simulink model "SVOC_DFIG"  (R2013a)
settings: Solver=ode15s  StartTime=0.0  StopTime=12  RelTol=1e-3
undefined symbols (not defined in the file): Cdc, Fb, Fs, Fsampling, Grid_Angle_init, Ibase, J_SCIG, Ki, Kp, Lgrid, Llr, Lls, Lm, Ls, Omegamech, P, Qgsc_ref, Qs_ref, Rr, Rs, Sbase, Trated, Ts, Vbase, Vdc_ref, Vp
libraries: powerlib x29, simulink_extras x5, powerlib_extras x5, simulink x4
(part 1 of 2)
settings Model: Creator=Sony  LastModifiedBy=Sony
settings DebuggingCC: UnconnectedInputMsg=none  UnconnectedOutputMsg=none  UnconnectedLineMsg=none

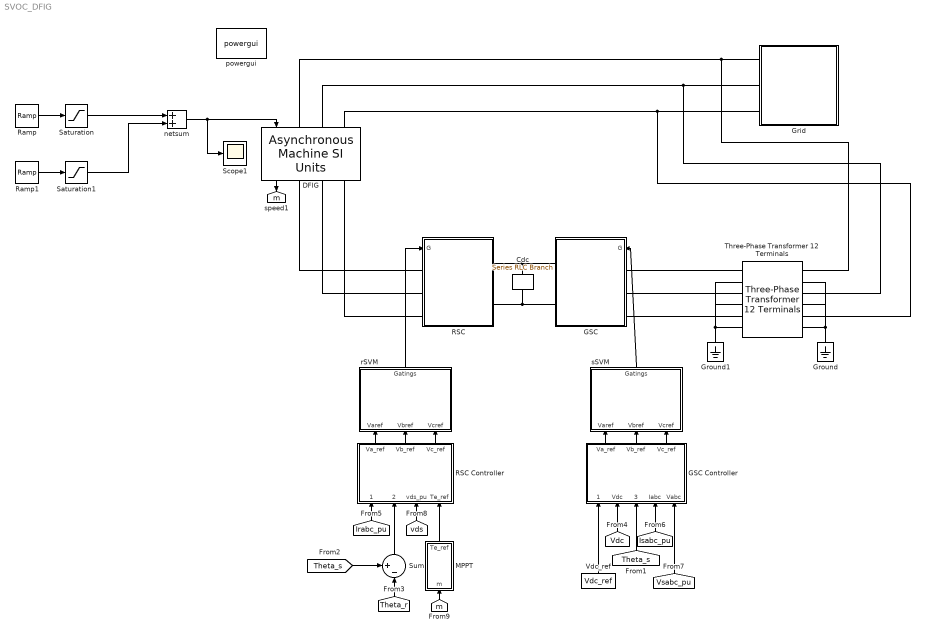
== system SVOC_DFIG ==
  Cdc : powerlib/Elements/Series RLC Branch  LConnTagsString=__new0  RConnTagsString=__new0  BranchType=C  Resistance=1e6  Inductance=1e-3  SetiL0=off  InitialCurrent=0  Capacitance=Cdc  Setx0=on  InitialVoltage=Vdc_ref*Vbase  Measurements=None
  DFIG : powerlib/Machines/Asynchronous Machine SI Units  PresetModel=No  MechanicalLoad=Speed w  ShowDetailedParameters=on  RotorType=Wound  ReferenceFrame=Synchronous  NominalParameters=[Sbase 690 50]  Stator=[Rs Lls]  Rotor=[Rr Llr]  Cage1=[ 0.022 0.226/377]  Cage2=[ 0.022 0.226/377]  Lm=Lm  Mechanical=[J_SCIG 0 P]  PolePairs=2  InitialConditions=[-5.86974e-12 0 317.758 317.758 317.758 -89.9144 150.086 30.0856]  Units=SI  LoadFlowParameters=-0.001  SimulateSaturation=off  Saturation=[0 0;0 0]  TsPowergui=0  TsBlock=-1  IterativeModel=Forward Euler  Pmec=1.5e6
  GSC : Subsystem
  GSC Controller : Subsystem
  Grid : Subsystem
  Ground : powerlib/Elements/Ground  LConnTagsString=a
  Ground1 : powerlib/Elements/Ground  LConnTagsString=a
  MPPT : Subsystem
  RSC : Subsystem
  RSC Controller : Subsystem
  Ramp : simulink/Sources/Ramp  slope=15  start=3  X0=1500*(2*pi/60)
  Ramp1 : simulink/Sources/Ramp  slope=-15  start=6  X0=0
  Saturation : Saturate  UpperLimit=1750*(2*pi/60)  LowerLimit=1225*(2*pi/60)
  Saturation1 : Saturate  UpperLimit=1750*(2*pi/60)  LowerLimit=-(1775-1225)*(2*pi/60)
  Scope1 : Scope
      settings: YMin=-50000  YMax=0  SaveName=ScopeData42
  Sum : Sum  Inputs=+-|
  Three-Phase Transformer 12 Terminals : powerlib/Elements/Three-Phase Transformer 12 Terminals  RatedPower=[ 1.5e6 50 ]  Winding1="[ Vbase*0.358 0.00001  0 ]"  Winding2=[ Vbase 0.00001 0]  RmXm=[ 1e6 1e6 ]
  Vdc_ref : Constant  Value=Vdc_ref
  netsum : Sum  Inputs=2  SaturateOnIntegerOverflow=on  InputSameDT=on  OutDataTypeStr=Inherit: Same as first input
  powergui : powerlib/powergui  Priority=1  SimulationMode=Continuous  SolverType=Tustin  SampleTime=1e-6  frequency=60  SPID=on  DisableSnubberDevices=off  DisableRonSwitches=off  DisableVfSwitches=off  SwTol=0  Interpol=off  DisplayEquations=on  frequencyindice=50  Pbase=1.5e6  ErrMax=1e-4  Iterations=50  UnitsV=kV  UnitsW=MW  FunctionMessages=on  echomessages=off  HookPort=off  EnableUseOfTLC=off  x0status=blocks  RestoreLinks=warning  ResistiveCurrentMeasurement=off  Frange=[0:2:500]  Ylog=off  Xlog=on  ShowGrid=off  save=off  variable=ZData  ZoomFFT=off  StartTime=0.0  cycles=1  DisplayStyle=1  fundamental=60  FreqAxis=off  MaxFrequency=1000  frequencyindicesteady=1  RmsSteady=1  display=off  Ts=0  methode=off
  rSVM : Subsystem
  sSVM : Subsystem
  tag scope: m=global
  wires:
  Vdc_ref/1 -> GSC Controller/1(Vdc_ref)
  [Vdc] -> GSC Controller/2(Vdc)
  GSC Controller/1(Va_ref) -> sSVM/1(Varef)
  GSC Controller/2(Vb_ref) -> sSVM/2(Vbref)
  GSC Controller/3(Vc_ref) -> sSVM/3(Vcref)
  [Theta_s] -> GSC Controller/3(Theta_s)
  sSVM/1(Gatings) -> GSC/1(G)
  rSVM/1(Gatings) -> RSC/1(G)
  RSC Controller/1(Va_ref) -> rSVM/1(Varef)
  RSC Controller/2(Vb_ref) -> rSVM/2(Vbref)
  RSC Controller/3(Vc_ref) -> rSVM/3(Vcref)
  Sum/1 -> RSC Controller/2(Theta_sl)
  [Theta_r] -> Sum/2
  DFIG/1 -> [m]
  [Isabc_pu] -> GSC Controller/4(Iabc)
  [Vsabc_pu] -> GSC Controller/5(Vabc)
  Saturation/1 -> netsum/1
  [Irabc_pu] -> RSC Controller/1(Irabc_pu)
  [vds] -> RSC Controller/3(vds_pu)
  MPPT/1(Te_ref) -> RSC Controller/4(Te_ref)
  [m] -> MPPT/1(m)
  [Theta_s] -> Sum/1
  Ramp/1 -> Saturation/1
  Ramp1/1 -> Saturation1/1
  Saturation1/1 -> netsum/2
  netsum/1 -> Scope1/1, DFIG/1
  connections:
  Grid/LConn1 -- DFIG/LConn1 -- Three-Phase Transformer 12 Terminals/RConn1
  Grid/LConn3 -- DFIG/LConn3 -- Three-Phase Transformer 12 Terminals/RConn5
  Grid/LConn2 -- DFIG/LConn2 -- Three-Phase Transformer 12 Terminals/RConn3
  RSC/LConn1 -- DFIG/RConn1
  RSC/LConn2 -- DFIG/RConn2
  RSC/LConn3 -- DFIG/RConn3
  GSC/RConn1 -- Cdc/LConn1 -- RSC/RConn1
  GSC/RConn2 -- Cdc/RConn1 -- RSC/RConn2
  GSC/LConn1 -- Three-Phase Transformer 12 Terminals/LConn1
  GSC/LConn2 -- Three-Phase Transformer 12 Terminals/LConn3
  GSC/LConn3 -- Three-Phase Transformer 12 Terminals/LConn5
  Three-Phase Transformer 12 Terminals/RConn6 -- Three-Phase Transformer 12 Terminals/RConn2 -- Three-Phase Transformer 12 Terminals/RConn4 -- Ground/LConn1
  Three-Phase Transformer 12 Terminals/LConn6 -- Three-Phase Transformer 12 Terminals/LConn2 -- Three-Phase Transformer 12 Terminals/LConn4 -- Ground1/LConn1

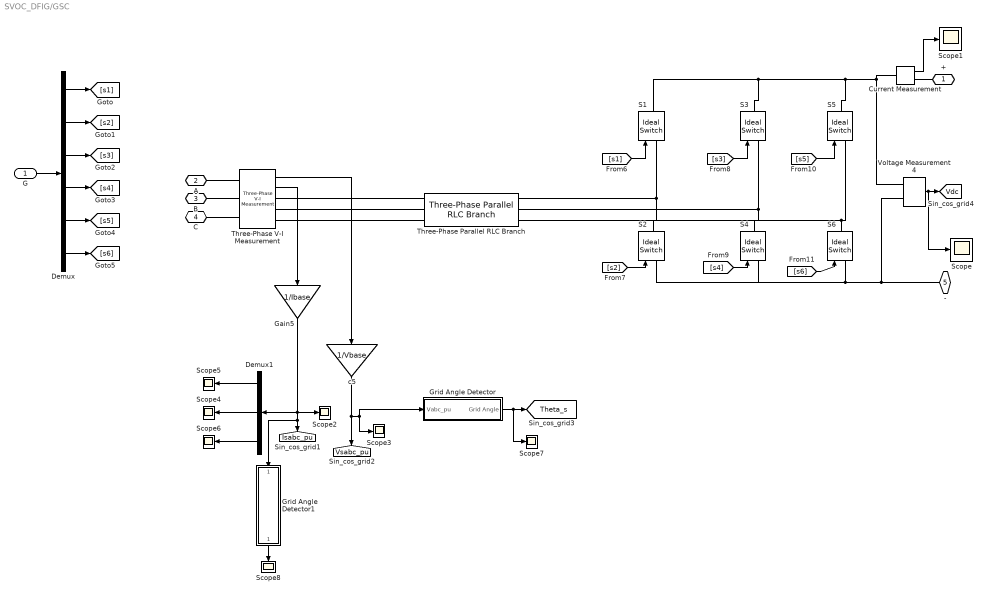
== system SVOC_DFIG/GSC ==
  G : Inport
  " S1" : powerlib/Power Electronics/Ideal Switch  Ron=Ron  Lon=0  IC=1  Rs=inf  Cs=inf  Measurements=off
  " S2" : powerlib/Power Electronics/Ideal Switch  Ron=Ron  Lon=0  IC=0  Rs=inf  Cs=inf  Measurements=off
  " S3" : powerlib/Power Electronics/Ideal Switch  Ron=Ron  Lon=0  IC=1  Rs=inf  Cs=inf  Measurements=off
  " S4" : powerlib/Power Electronics/Ideal Switch  Ron=Ron  Lon=0  IC=0  Rs=inf  Cs=inf  Measurements=off
  " S5" : powerlib/Power Electronics/Ideal Switch  Ron=Ron  Lon=0  IC=1  Rs=inf  Cs=inf  Measurements=off
  " S6" : powerlib/Power Electronics/Ideal Switch  Ron=Ron  Lon=0  IC=0  Rs=inf  Cs=inf  Measurements=off
  Current Measurement : powerlib/Measurements/Current Measurement  PhasorSimulation=off  OutputType=Complex  PSBequivalent=0
  Demux : Demux  Outputs=6
  Demux1 : Demux  Outputs=3
  Gain5 : Gain  Gain=1/Ibase
  Grid Angle Detector : Subsystem
  Grid Angle Detector1 : Subsystem
  Scope{,1..8} (9 alike) : Scope
      Scope settings: YMin=0  YMax=600  SaveName=ScopeData8
      Scope1 settings: YMin=-225  YMax=200  SaveName=ScopeData9
      Scope2 settings: YMin=-50  YMax=50  SaveName=ScopeData33
      Scope3 settings: SaveName=ScopeData32
      Scope4 settings: SaveName=ScopeData14
      Scope5 settings: YMin=-2000  YMax=2500  SaveName=ScopeData39
      Scope6 settings: SaveName=ScopeData19
      Scope7 settings: YMin=0  YMax=6.5  SaveName=ScopeData27
      Scope8 settings: YMin=0  YMax=6.5  SaveName=ScopeData54
  Three-Phase Parallel RLC Branch : powerlib/Elements/Three-Phase Parallel RLC Branch  LConnTagsString=A|B|C  RConnTagsString=A|B|C  BranchType=L  Resistance=inf  Inductance=Lgrid  Capacitance=1e-6  Measurements=None
  Three-Phase V-I Measurement : powerlib/Measurements/Three-Phase V-I Measurement  VoltageMeasurement=phase-to-ground  SetLabelV=off  LabelV=Vabc  Vpu=off  VpuLL=off  CurrentMeasurement=yes  SetLabelI=off  LabelI=Iabc  Ipu=off  Pbase=100e6  Vbase=500e3  OutputType=Complex  PhasorSimulation=off  PSBequivalent=0
  Voltage Measurement4 : powerlib/Measurements/Voltage Measurement  PhasorSimulation=off  OutputType=Complex  PSBequivalent=0
  c5 : Gain  Gain=1/Vbase
  + : PMIOPort  Port=1  Side=Right
  A : PMIOPort  Port=2  Side=Left
  B : PMIOPort  Port=3  Side=Left
  C : PMIOPort  Port=4  Side=Left
  - : PMIOPort  Port=5  Side=Right
  tag scope: Isabc_pu=global, Theta_s=global, Vdc=global, Vsabc_pu=global
  wires:
  [s1] -> " S1"/1
  [s5] -> " S5"/1
  Demux/1 -> [s1]
  Demux/2 -> [s2]
  Demux/3 -> [s3]
  Demux/4 -> [s4]
  Demux/5 -> [s5]
  Demux/6 -> [s6]
  G/1 -> Demux/1
  [s3] -> " S3"/1
  Grid Angle Detector/1(Grid Angle) -> Scope7/1, [Theta_s]
  Voltage Measurement4/1 -> Scope/1, [Vdc]
  [s6] -> " S6"/1
  [s4] -> " S4"/1
  [s2] -> " S2"/1
  Gain5/1 -> Scope2/1, Grid Angle Detector1/1(Vabc_pu), [Isabc_pu], Demux1/1
  c5/1 -> Scope3/1, Grid Angle Detector/1(Vabc_pu), [Vsabc_pu]
  Demux1/1 -> Scope5/1
  Demux1/2 -> Scope4/1
  Demux1/3 -> Scope6/1
  Current Measurement/1 -> Scope1/1
  Grid Angle Detector1/1(Grid Angle) -> Scope8/1
  Three-Phase V-I Measurement/1 -> c5/1
  Three-Phase V-I Measurement/2 -> Gain5/1
  connections:
  Voltage Measurement4/LConn1 -- Current Measurement/LConn1 -- " S5"/RConn1 -- " S3"/RConn1 -- " S1"/RConn1
  " S2"/RConn1 -- " S1"/LConn1 -- Three-Phase Parallel RLC Branch/RConn1
  " S4"/RConn1 -- " S3"/LConn1 -- Three-Phase Parallel RLC Branch/RConn2
  -/RConn1 -- Voltage Measurement4/LConn2 -- " S2"/LConn1 -- " S4"/LConn1 -- " S6"/LConn1
  A/RConn1 -- Three-Phase V-I Measurement/LConn1
  B/RConn1 -- Three-Phase V-I Measurement/LConn2
  C/RConn1 -- Three-Phase V-I Measurement/LConn3
  " S6"/RConn1 -- " S5"/LConn1 -- Three-Phase Parallel RLC Branch/RConn3
  Current Measurement/RConn1 -- +/RConn1
  Three-Phase Parallel RLC Branch/LConn1 -- Three-Phase V-I Measurement/RConn1
  Three-Phase Parallel RLC Branch/LConn2 -- Three-Phase V-I Measurement/RConn2
  Three-Phase Parallel RLC Branch/LConn3 -- Three-Phase V-I Measurement/RConn3

== system SVOC_DFIG/GSC Controller ==
  Vdc_ref : Inport
  Vdc : Inport  Port=2
  Theta_s : Inport  Port=3
  Iabc : Inport  Port=4
  Vabc : Inport  Port=5
  Add : Sum  Inputs=+-
  Add1 : Sum  Inputs=-+-
  Add2 : Sum  Inputs=-++
  Constant : Constant  Value=Qgsc_ref
  Mux6 : Mux  Inputs=2
  Product1 : Product  Inputs=*/
  Scope{1,3..5} (4 alike) : Scope  NumInputPorts=4
      Scope1 settings: YMin=0.506283~-1~-3~-3  YMax=0.506296~1~2.5~3  SaveName=ScopeData47
      Scope3 settings: YMin=1.04021~1.04021~-3~-6.05  YMax=1.14971~1.14971~3~-5.75  SaveName=ScopeData23
      Scope4 settings: YMin=-27.475~-75~-90~890  YMax=-27.275~75~40~1020  SaveName=ScopeData38
      Scope5 settings: YMin=-1~-20~-20~-2.5  YMax=1~20~20~2  SaveName=ScopeData43
  Sum : Sum  Inputs=|+-
  Sum2 : Sum  Inputs=|+-
  Vdc_Ctr1 : powerlib_extras/Discrete  Control Blocks/Discrete PI Controller  Kp=Kp  Ki=Ki  Par_Limits=[1e6 -1e6]  Init=0  Ts=50e-6
  Xl1 : Subsystem
  Xl2 : Subsystem
  abc/dq : Subsystem
  abc/dq1 : Subsystem
  constant2 : Gain  Gain=(1/Vbase)
  constant5 : Gain  Gain=-1.5
  dq/abc : Subsystem
  id_Ctr1 : powerlib_extras/Discrete  Control Blocks/Discrete PI Controller  Kp=Kp  Ki=Ki  Par_Limits=[1e6 -1e6]  Init=0  Ts=50e-6
  iq_Ctr2 : powerlib_extras/Discrete  Control Blocks/Discrete PI Controller  Kp=Kp  Ki=Ki  Par_Limits=[1e6 -1e6]  Init=0  Ts=50e-6
  Va_ref : Outport
  Vb_ref : Outport  Port=2
  Vc_ref : Outport  Port=3
  tag scope: vds=global
  wires:
  Vdc_ref/1 -> Scope3/1, Add/1
  Add/1 -> Vdc_Ctr1/1, Scope3/3
  constant5/1 -> Product1/2
  Constant/1 -> Product1/1
  dq/abc/1(Va) -> Va_ref/1
  dq/abc/2(Vb) -> Vb_ref/1
  dq/abc/3(Vc) -> Vc_ref/1
  Mux6/1 -> dq/abc/1(vdq)
  id_Ctr1/1 -> Scope4/4, Add2/1
  Sum/1 -> Scope4/3, id_Ctr1/1
  abc/dq/2(Vqg) -> Scope1/2, Add1/2
  abc/dq/1(Vdg) -> Add2/2, constant5/1, Scope1/1, [vds]
  Sum2/1 -> Scope5/3, iq_Ctr2/1
  Xl2/1(Out1) -> Add1/3
  Theta_s/1 -> abc/dq1/2(Theta), abc/dq/2(Theta), dq/abc/2(Theta)
  Xl1/1(Out1) -> Add2/3
  Iabc/1 -> abc/dq1/1(Iabc)
  Vabc/1 -> abc/dq/1(Vabc)
  Add2/1 -> Mux6/1
  Add1/1 -> Mux6/2
  constant2/1 -> Scope3/2, Add/2
  abc/dq1/1(Idg) -> Scope1/3, Xl2/1(In1), Scope4/2, Sum/2
  Product1/1 -> Scope5/1, Sum2/1
  abc/dq1/2(Iqg) -> Xl1/1(In1), Scope1/4, Scope5/2, Sum2/2
  Vdc_Ctr1/1 -> Scope4/1, Sum/1, Scope3/4
  iq_Ctr2/1 -> Scope5/4, Add1/1
  Vdc/1 -> constant2/1

== system SVOC_DFIG/Grid ==
  AC Voltage Source1 : powerlib/Electrical Sources/AC Voltage Source  Amplitude=Vp  Phase=-120+Grid_Angle_init  Frequency=50  SampleTime=0  Measurements=None
  AC Voltage Source2 : powerlib/Electrical Sources/AC Voltage Source  Amplitude=Vp  Phase=-240+Grid_Angle_init  Frequency=50  SampleTime=0  Measurements=None
  AC Voltage Source3 : powerlib/Electrical Sources/AC Voltage Source  Amplitude=Vp  Phase=0+Grid_Angle_init  Frequency=50  SampleTime=0  Measurements=None
  Demux1 : Demux  Outputs=3
  Demux2 : Demux  Outputs=3
  Gain5 : Gain  Gain=1/Ibase
  Grid Angle Detector : Subsystem
  Ground : powerlib/Elements/Ground  LConnTagsString=a
  Scope{1..10} (10 alike) : Scope
      Scope1 settings: YMin=-0.35  YMax=0.025  SaveName=ScopeData36
      Scope2 settings: YMin=-50  YMax=50  SaveName=ScopeData21
      Scope3 settings: YMin=-1.5  YMax=1.5  SaveName=ScopeData35
      Scope4 settings: SaveName=ScopeData48
      Scope5 settings: SaveName=ScopeData49
      Scope6 settings: YMin=-15  YMax=15  SaveName=ScopeData50
      Scope7 settings: SaveName=ScopeData51
      Scope8 settings: SaveName=ScopeData52
      Scope9 settings: YMin=-1.5  YMax=1.5  SaveName=ScopeData53
  Three-Phase V-I Measurement : powerlib/Measurements/Three-Phase V-I Measurement  VoltageMeasurement=phase-to-ground  SetLabelV=off  LabelV=Vabc  Vpu=off  VpuLL=off  CurrentMeasurement=yes  SetLabelI=off  LabelI=Iabc  Ipu=off  Pbase=100e6  Vbase=500e3  OutputType=Complex  PhasorSimulation=off  PSBequivalent=0
  c5 : Gain  Gain=1/Vbase
  Phase A : PMIOPort  Port=1  Side=Left
  Phase B : PMIOPort  Port=2  Side=Left
  Phase C : PMIOPort  Port=3  Side=Left
  tag scope: iag=global, vag=global
  wires:
  Grid Angle Detector/1(Grid Angle) -> Scope1/1
  Gain5/1 -> Demux1/1, Scope2/1
  Three-Phase V-I Measurement/2 -> Gain5/1
  Three-Phase V-I Measurement/1 -> Grid Angle Detector/1(Vabc_pu), c5/1, Scope3/1
  Demux1/1 -> [iag], Scope6/1
  Demux1/2 -> Scope5/1
  Demux1/3 -> Scope7/1
  c5/1 -> Demux2/1, Scope4/1
  Demux2/1 -> [vag], Scope9/1
  Demux2/2 -> Scope8/1
  Demux2/3 -> Scope10/1
  connections:
  Three-Phase V-I Measurement/LConn1 -- AC Voltage Source3/RConn1
  Three-Phase V-I Measurement/LConn3 -- AC Voltage Source2/RConn1
  AC Voltage Source2/LConn1 -- AC Voltage Source3/LConn1 -- AC Voltage Source1/LConn1 -- Ground/LConn1
  Phase A/RConn1 -- Three-Phase V-I Measurement/RConn1
  Phase B/RConn1 -- Three-Phase V-I Measurement/RConn2
  Phase C/RConn1 -- Three-Phase V-I Measurement/RConn3
  AC Voltage Source1/RConn1 -- Three-Phase V-I Measurement/LConn2

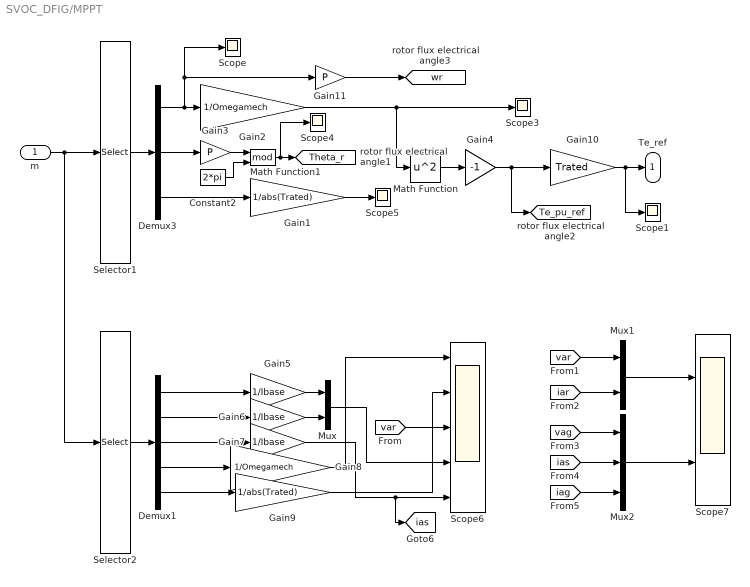
== system SVOC_DFIG/MPPT ==
  m : Inport
  Constant2 : Constant  Value=2*pi
  Demux1 : Demux  Outputs=5
  Demux3 : Demux  Outputs=3
  Gain1 : Gain  Gain=1/abs(Trated)
  Gain10 : Gain  Gain=Trated
  Gain11 : Gain  Gain=P
  Gain2 : Gain  Gain=1/Omegamech  SampleTime=1/Fsampling
  Gain3 : Gain  Gain=P
  Gain4 : Gain  Gain=-1
  Gain5 : Gain  Gain=1/Ibase
  Gain6 : Gain  Gain=1/Ibase
  Gain7 : Gain  Gain=1/Ibase
  Gain8 : Gain  Gain=1/Omegamech  SampleTime=1/Fsampling
  Gain9 : Gain  Gain=1/abs(Trated)
  Math Function : Math  Operator=square  SaturateOnIntegerOverflow=on
  Math Function1 : Math  Operator=mod  SampleTime=1/Fsampling  SaturateOnIntegerOverflow=on
  Mux : Mux  Inputs=2
  Mux1 : Mux  Inputs=2
  Mux2 : Mux  Inputs=3
  Scope{,1,3..5} (5 alike) : Scope
      Scope settings: YMin=127.5  YMax=185  SaveName=ScopeData4
      Scope1 settings: YMin=-9010.65  YMax=-3010.65  SaveName=ScopeData7
      Scope3 settings: YMin=0.4  YMax=1.2  SaveName=ScopeData15
      Scope4 settings: YMin=0  YMax=6.5  SaveName=ScopeData17
      Scope5 settings: YMin=-10  YMax=10  SaveName=ScopeData18
  Scope6 : Scope  NumInputPorts=5
      settings: YMin=0.6~-5~-1.25~-5~-5  YMax=1.2~5~1.25~5~5  SaveName=ScopeData28
  Scope7 : Scope  NumInputPorts=2
      settings: YMin=-2~-2  YMax=2~2  SaveName=ScopeData55
  Selector1 : Selector  InputPortWidth=22  IndexOptions=Index vector (dialog)  Indices=[20 22 21]  OutputSizes=1
  Selector2 : Selector  InputPortWidth=22  IndexOptions=Index vector (dialog)  Indices=[1 2 11 20 21]  OutputSizes=1
  Te_ref : Outport
  tag scope: Te_pu_ref=global, Theta_r=global, ias=global, wr=global
  wires:
  Demux3/3 -> Gain1/1
  Selector1/1 -> Demux3/1
  Gain2/1 -> Math Function/1, Scope3/1
  Constant2/1 -> Math Function1/2
  Demux3/2 -> Gain3/1
  Math Function/1 -> Gain4/1
  Gain10/1 -> Scope1/1, Te_ref/1
  Gain3/1 -> Math Function1/1
  Math Function1/1 -> Scope4/1, [Theta_r]
  Gain1/1 -> Scope5/1
  Selector2/1 -> Demux1/1
  m/1 -> Selector2/1, Selector1/1
  Demux1/1 -> Gain5/1
  Demux1/2 -> Gain6/1
  Demux1/3 -> Gain7/1
  Demux1/4 -> Gain8/1
  Demux1/5 -> Gain9/1
  Gain4/1 -> [Te_pu_ref], Gain10/1
  Gain7/1 -> [ias], Scope6/5
  Gain5/1 -> Mux/1
  Gain6/1 -> Mux/2
  Mux/1 -> Scope6/4
  [var] -> Scope6/3
  Gain8/1 -> Scope6/1
  Gain9/1 -> Scope6/2
  Mux1/1 -> Scope7/1
  Mux2/1 -> Scope7/2
  Demux3/1 -> Scope/1, Gain11/1, Gain2/1
  Gain11/1 -> [wr]
  [var] -> Mux1/1
  [iar] -> Mux1/2
  [ias] -> Mux2/2
  [iag] -> Mux2/3
  [vag] -> Mux2/1

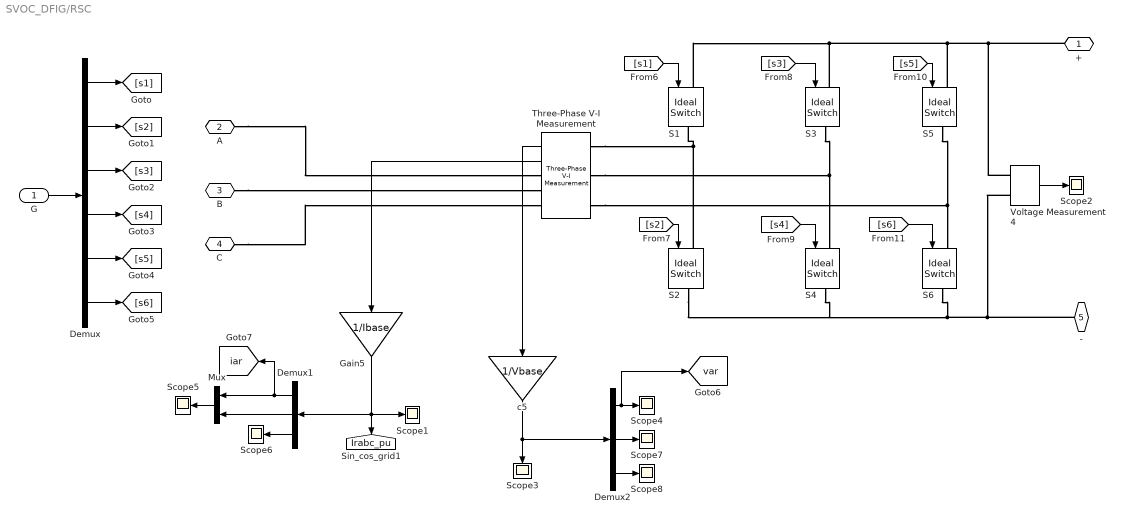
== system SVOC_DFIG/RSC ==
  G : Inport
  " S1" : powerlib/Power Electronics/Ideal Switch  Ron=Ron  Lon=0  IC=1  Rs=inf  Cs=inf  Measurements=off
  " S2" : powerlib/Power Electronics/Ideal Switch  Ron=Ron  Lon=0  IC=0  Rs=inf  Cs=inf  Measurements=off
  " S3" : powerlib/Power Electronics/Ideal Switch  Ron=Ron  Lon=0  IC=1  Rs=inf  Cs=inf  Measurements=off
  " S4" : powerlib/Power Electronics/Ideal Switch  Ron=Ron  Lon=0  IC=0  Rs=inf  Cs=inf  Measurements=off
  " S5" : powerlib/Power Electronics/Ideal Switch  Ron=Ron  Lon=0  IC=1  Rs=inf  Cs=inf  Measurements=off
  " S6" : powerlib/Power Electronics/Ideal Switch  Ron=Ron  Lon=0  IC=0  Rs=inf  Cs=inf  Measurements=off
  Demux : Demux  Outputs=6
  Demux1 : Demux  Outputs=3
  Demux2 : Demux  Outputs=3
  Gain5 : Gain  Gain=1/Ibase
  Mux : Mux  Inputs=2
  Scope{1..8} (8 alike) : Scope
      Scope1 settings: YMin=-25  YMax=22.5  SaveName=ScopeData31
      Scope2 settings: YMin=0  YMax=570.102
      Scope3 settings: YMin=-2  YMax=2  SaveName=ScopeData30
      Scope4 settings: YMin=-2  YMax=2  SaveName=ScopeData41
      Scope5 settings: YMin=-15  YMax=15  SaveName=ScopeData40
      Scope6 settings: SaveName=ScopeData20
      Scope7 settings: SaveName=ScopeData24
      Scope8 settings: SaveName=ScopeData25
  Three-Phase V-I Measurement : powerlib/Measurements/Three-Phase V-I Measurement  VoltageMeasurement=phase-to-ground  SetLabelV=off  LabelV=Vabc  Vpu=off  VpuLL=off  CurrentMeasurement=yes  SetLabelI=off  LabelI=Iabc  Ipu=off  Pbase=100e6  Vbase=500e3  OutputType=Complex  PhasorSimulation=off  PSBequivalent=0
  Voltage Measurement4 : powerlib/Measurements/Voltage Measurement  PhasorSimulation=off  OutputType=Complex  PSBequivalent=0
  c5 : Gain  Gain=1/Vbase
  + : PMIOPort  Port=1  Side=Right
  A : PMIOPort  Port=2  Side=Left
  B : PMIOPort  Port=3  Side=Left
  C : PMIOPort  Port=4  Side=Left
  - : PMIOPort  Port=5  Side=Right
  tag scope: Irabc_pu=global, iar=global, var=global
  wires:
  [s1] -> " S1"/1
  [s5] -> " S5"/1
  Demux/1 -> [s1]
  Demux/2 -> [s2]
  Demux/3 -> [s3]
  Demux/4 -> [s4]
  Demux/5 -> [s5]
  Demux/6 -> [s6]
  G/1 -> Demux/1
  [s2] -> " S2"/1
  [s3] -> " S3"/1
  [s4] -> " S4"/1
  [s6] -> " S6"/1
  Voltage Measurement4/1 -> Scope2/1
  Three-Phase V-I Measurement/1 -> c5/1
  Gain5/1 -> Scope1/1, [Irabc_pu], Demux1/1
  Demux1/1 -> [iar], Mux/1
  Demux1/2 -> Mux/2
  Mux/1 -> Scope5/1
  c5/1 -> Demux2/1, Scope3/1
  Demux2/1 -> [var], Scope4/1
  Demux1/3 -> Scope6/1
  Demux2/2 -> Scope7/1
  Demux2/3 -> Scope8/1
  Three-Phase V-I Measurement/2 -> Gain5/1
  connections:
  +/RConn1 -- Voltage Measurement4/LConn1 -- " S5"/LConn1 -- " S3"/LConn1 -- " S1"/LConn1
  " S2"/LConn1 -- " S1"/RConn1 -- Three-Phase V-I Measurement/LConn1
  " S3"/RConn1 -- " S4"/LConn1 -- Three-Phase V-I Measurement/LConn2
  " S5"/RConn1 -- " S6"/LConn1 -- Three-Phase V-I Measurement/LConn3
  -/RConn1 -- Voltage Measurement4/LConn2 -- " S2"/RConn1 -- " S4"/RConn1 -- " S6"/RConn1
  A/RConn1 -- Three-Phase V-I Measurement/RConn1
  B/RConn1 -- Three-Phase V-I Measurement/RConn2
  C/RConn1 -- Three-Phase V-I Measurement/RConn3

== system SVOC_DFIG/RSC Controller ==
  note: actual value
  Irabc_pu : Inport
  Theta_sl : Inport  Port=2
  vds_pu : Inport  Port=3
  Te_ref : Inport  Port=4
  Gain : Gain  Gain=(2*Ls*Qs_ref)/(3*Lm)
  Gain1 : Gain  Gain=1/(2*pi*Fb*Lm)
  Gain2 : Gain  Gain=-(2*2*pi*Fb*Ls)/(3*P*Lm)
  Gain3 : Gain  Gain=Vbase
  Gain4 : Gain  Gain=1/Ibase
  Gain5 : Gain  Gain=1/Ibase
  Math Function : Math  Operator=reciprocal  SaturateOnIntegerOverflow=on
  Math Function1 : Math  Operator=reciprocal  SaturateOnIntegerOverflow=on
  Multiply : Product
  Scope2 : Scope  NumInputPorts=4
      settings: YMin=-1~-1~-1~-0.5  YMax=1~1~1~1.25  SaveName=ScopeData44
  Scope3 : Scope  NumInputPorts=4
      settings: YMin=2.56425~2.51~-0.03~-0.005  YMax=2.56433~2.59~0.05~0.055  SaveName=ScopeData16
  Sum1 : Sum  Inputs=-+|
  Sum2 : Sum  Inputs=-+|
  Sum3 : Sum  Inputs=-+|
  abc/dq1 : Subsystem
  dq/abc : Subsystem
  id_Ctr1 : powerlib_extras/Discrete  Control Blocks/Discrete PI Controller  Kp=Kp  Ki=Ki  Par_Limits=[1e6 -1e6]  Init=0  Ts=50e-6
  id_Ctr2 : powerlib_extras/Discrete  Control Blocks/Discrete PI Controller  Kp=Kp  Ki=Ki  Par_Limits=[1e6 -1e6]  Init=0  Ts=50e-6
  Va_ref : Outport
  Vb_ref : Outport  Port=2
  Vc_ref : Outport  Port=3
  wires:
  dq/abc/3(Vcr_ref) -> Vc_ref/1
  Sum1/1 -> id_Ctr2/1, Scope2/3
  Math Function1/1 -> Gain2/1
  Sum2/1 -> Scope3/3, id_Ctr1/1
  Gain3/1 -> Gain1/1, Math Function1/1, Math Function/1
  dq/abc/2(Vbr_ref) -> Vb_ref/1
  id_Ctr2/1 -> Scope2/4, dq/abc/2(vq_ref)
  Gain1/1 -> Sum3/1
  id_Ctr1/1 -> Scope3/4, dq/abc/1(vd_ref)
  Gain/1 -> Sum3/2
  Math Function/1 -> Gain/1
  Te_ref/1 -> Multiply/2
  Gain2/1 -> Multiply/1
  Irabc_pu/1 -> abc/dq1/1(Irabc)
  dq/abc/1(Var_ref) -> Va_ref/1
  Theta_sl/1 -> abc/dq1/2(Theta_sl), dq/abc/3(Theta_sl)
  abc/dq1/1(Idr) -> Scope3/2, Sum2/1
  abc/dq1/2(Iqr) -> Scope2/2, Sum1/1
  Gain5/1 -> Sum2/2, Scope3/1
  Gain4/1 -> Sum1/2, Scope2/1
  vds_pu/1 -> Gain3/1
  Sum3/1 -> Gain4/1
  Multiply/1 -> Gain5/1

== system SVOC_DFIG/rSVM ==
  Varef : Inport
  Vbref : Inport  Port=2
  Vcref : Inport  Port=3
  Add : Sum
  Cartesian to Polar : simulink_extras/Transformations/Cartesian to Polar
  Constant : Constant  Value=2*pi
  Constant1 : Constant  Value=2*pi
  Divide : Product  Inputs=/*
  Dwell Time Calculator : Subsystem
  Math Function : Math  Operator=rem  SaturateOnIntegerOverflow=on
  Mux7 : Mux  Inputs=3
  Pulses : Subsystem
  Saturation : Saturate  UpperLimit=1  LowerLimit=0.01  SampleTime=1/Fsampling
  Sector judge : Subsystem
  Ts : Constant  Value=Ts
  Zero-Order Hold : ZeroOrderHold  SampleTime=Ts/2
  Zero-Order Hold1 : ZeroOrderHold  SampleTime=Ts/2
  abc/alphabeta : Subsystem
  constant : Gain  Gain=3^0.5
  constant2 : Gain  Gain=(1/Vbase)
  ma : Scope
      settings: SaveName=ScopeData5
  theta : Scope
      settings: YMin=0  YMax=6.5  SaveName=ScopeData6
  Gatings : Outport
  wires:
  Dwell Time Calculator/3(T0) -> Pulses/4(T0)
  constant/1 -> Divide/2
  Pulses/1(Gating) -> Gatings/1
  Cartesian to Polar/1 -> constant/1
  Divide/1 -> Saturation/1
  Ts/1 -> Dwell Time Calculator/3(Ts)
  Varef/1 -> Mux7/1
  Dwell Time Calculator/1(Ta) -> Pulses/2(Ta1)
  Dwell Time Calculator/2(Tb) -> Pulses/3(Tb1)
  Sector judge/2(Cal_theta) -> Dwell Time Calculator/1(Theta)
  Saturation/1 -> Zero-Order Hold/1, ma/1
  Zero-Order Hold/1 -> Dwell Time Calculator/2(ma)
  Zero-Order Hold1/1 -> Sector judge/1(theta), theta/1
  Sector judge/1(Sector) -> Pulses/1(Sector)
  abc/alphabeta/1(Valpha) -> Cartesian to Polar/1
  Mux7/1 -> abc/alphabeta/1(Vabc)
  Vbref/1 -> Mux7/2
  abc/alphabeta/2(Vbeta) -> Cartesian to Polar/2
  Vcref/1 -> Mux7/3
  Cartesian to Polar/2 -> Add/1
  Math Function/1 -> Zero-Order Hold1/1
  Constant/1 -> Add/2
  Add/1 -> Math Function/1
  Constant1/1 -> Math Function/2
  constant2/1 -> Divide/1
  [Vdc] -> constant2/1

== system SVOC_DFIG/sSVM ==
  Varef : Inport
  Vbref : Inport  Port=2
  Vcref : Inport  Port=3
  Add : Sum
  Cartesian to Polar : simulink_extras/Transformations/Cartesian to Polar
  Constant : Constant  Value=2*pi
  Constant1 : Constant  Value=2*pi
  Divide : Product  Inputs=/*
  Dwell Time Calculator : Subsystem
  Math Function : Math  Operator=rem  SaturateOnIntegerOverflow=on
  Mux7 : Mux  Inputs=3
  Pulses : Subsystem
  Saturation : Saturate  UpperLimit=1  LowerLimit=0.01  SampleTime=1/Fsampling
  Scope{,1..3} (4 alike) : Scope
      Scope settings: YMin=0  YMax=8  SaveName=ScopeData10
      Scope1 settings: YMin=25  YMax=350  SaveName=ScopeData37
      Scope2 settings: YMin=0  YMax=8  SaveName=ScopeData45
      Scope3 settings: YMin=-0.01  YMax=0.01  SaveName=ScopeData46
  Sector judge : Subsystem
  Ts : Constant  Value=Ts
  Zero-Order Hold : ZeroOrderHold  SampleTime=Ts/2
  Zero-Order Hold1 : ZeroOrderHold  SampleTime=Ts/2
  abc/alphabeta : Subsystem
  constant : Gain  Gain=3^0.5
  constant2 : Gain  Gain=(1/Vbase)
  ma : Scope
      settings: YMin=0  YMax=2  SaveName=ScopeData5
  theta : Scope
      settings: YMin=0  YMax=6.5  SaveName=ScopeData6
  Gatings : Outport
  wires:
  Dwell Time Calculator/3(T0) -> Pulses/4(T0)
  constant/1 -> Scope1/1, Divide/2
  Pulses/1(Gating) -> Gatings/1
  Cartesian to Polar/1 -> constant/1
  Divide/1 -> Scope3/1, Saturation/1
  Ts/1 -> Dwell Time Calculator/3(Ts)
  Varef/1 -> Mux7/1
  Dwell Time Calculator/1(Ta) -> Pulses/2(Ta1)
  Dwell Time Calculator/2(Tb) -> Pulses/3(Tb1)
  Sector judge/2(Cal_theta) -> Dwell Time Calculator/1(Theta)
  Saturation/1 -> Zero-Order Hold/1, ma/1
  Zero-Order Hold/1 -> Dwell Time Calculator/2(ma)
  constant2/1 -> Scope2/1, Divide/1
  Zero-Order Hold1/1 -> Sector judge/1(theta), theta/1
  Sector judge/1(Sector) -> Scope/1, Pulses/1(Sector)
  abc/alphabeta/1(Valpha) -> Cartesian to Polar/1
  Mux7/1 -> abc/alphabeta/1(Vabc)
  Vbref/1 -> Mux7/2
  abc/alphabeta/2(Vbeta) -> Cartesian to Polar/2
  Vcref/1 -> Mux7/3
  Cartesian to Polar/2 -> Add/1
  Math Function/1 -> Zero-Order Hold1/1
  Constant/1 -> Add/2
  Add/1 -> Math Function/1
  Constant1/1 -> Math Function/2
  [Vdc] -> constant2/1

== system SVOC_DFIG/GSC/Grid Angle Detector ==
  Vabc_pu : Inport
  Add : Sum
  Beta1 : Fcn  Expr=(1/(3^.5))*(u(1)+2*u(2))
  Cartesian to Polar1 : simulink_extras/Transformations/Cartesian to Polar
  Constant : Constant  Value=2*pi
  Math Function : Math  Operator=rem  SaturateOnIntegerOverflow=on
  Scope3 : Scope  NumInputPorts=2
      settings: YMin=-1~-5  YMax=2~5  SaveName=ScopeData34
  Scope5 : Scope
      settings: SaveName=ScopeData13
  alpha1 : Fcn  Expr=u(1)
  Grid Angle : Outport
  wires:
  Beta1/1 -> Scope3/2, Cartesian to Polar1/2
  Vabc_pu/1 -> alpha1/1, Beta1/1
  Math Function/1 -> Grid Angle/1
  alpha1/1 -> Scope3/1, Cartesian to Polar1/1
  Cartesian to Polar1/2 -> Add/1
  Constant/1 -> Math Function/2, Add/2
  Add/1 -> Math Function/1
  Cartesian to Polar1/1 -> Scope5/1

== system SVOC_DFIG/GSC/Grid Angle Detector1 ==
  Vabc_pu : Inport
  Add : Sum
  Beta1 : Fcn  Expr=(1/(3^.5))*(u(1)+2*u(2))
  Cartesian to Polar1 : simulink_extras/Transformations/Cartesian to Polar
  Constant : Constant  Value=2*pi
  Math Function : Math  Operator=rem  SaturateOnIntegerOverflow=on
  Scope3 : Scope  NumInputPorts=2
      settings: YMin=-1~-5  YMax=2~5  SaveName=ScopeData34
  Scope5 : Scope
      settings: SaveName=ScopeData13
  alpha1 : Fcn  Expr=u(1)
  Grid Angle : Outport
  wires:
  Beta1/1 -> Scope3/2, Cartesian to Polar1/2
  Vabc_pu/1 -> alpha1/1, Beta1/1
  Math Function/1 -> Grid Angle/1
  alpha1/1 -> Scope3/1, Cartesian to Polar1/1
  Cartesian to Polar1/2 -> Add/1
  Constant/1 -> Math Function/2, Add/2
  Add/1 -> Math Function/1
  Cartesian to Polar1/1 -> Scope5/1

== system SVOC_DFIG/GSC Controller/Xl1 ==
  In1 : Inport
  Constant1 : Constant  Value=2*pi*50
  Constant2 : Constant  Value=0
  Gain : Gain  Gain=Lgrid/Vbase
  Matrix Multiply : Product
  netsum : Sum  Inputs=-+  SaturateOnIntegerOverflow=on  InputSameDT=on  OutDataTypeStr=Inherit: Same as first input
  Out1 : Outport
  wires:
  In1/1 -> Matrix Multiply/1
  Matrix Multiply/1 -> Gain/1
  Constant2/1 -> netsum/1
  Constant1/1 -> netsum/2
  netsum/1 -> Matrix Multiply/2
  Gain/1 -> Out1/1

== system SVOC_DFIG/GSC Controller/Xl2 ==
  In1 : Inport
  Constant1 : Constant  Value=2*pi*50
  Constant2 : Constant  Value=0
  Gain : Gain  Gain=Lgrid/Vbase
  Matrix Multiply : Product
  netsum : Sum  Inputs=-+  SaturateOnIntegerOverflow=on  InputSameDT=on  OutDataTypeStr=Inherit: Same as first input
  Out1 : Outport
  wires:
  In1/1 -> Matrix Multiply/1
  Matrix Multiply/1 -> Gain/1
  Constant1/1 -> netsum/2
  netsum/1 -> Matrix Multiply/2
  Gain/1 -> Out1/1
  Constant2/1 -> netsum/1

== system SVOC_DFIG/GSC Controller/abc//dq ==
  Vabc : Inport
  Theta : Inport  Port=2
  Add{,1,3..4} (4 alike) : Sum  Inputs=+-
  Add2 : Sum  Inputs=+++
  Add5 : Sum  Inputs=+++
  Constant : Constant  Value=(2*pi)/3
  Constant1 : Constant  Value=(4*pi)/3
  Constant2 : Constant  Value=(2*pi)/3
  Constant3 : Constant  Value=(4*pi)/3
  Demux2 : Demux  Outputs=3
  Gain : Gain  Gain=2/3
  Gain1 : Gain  Gain=-(2/3)*0
  Product{1..6} (6 alike) : Product
  Scope5 : Scope  NumInputPorts=4
      settings: YMin=1.41421~-1~-1~-1  YMax=1.41421~1~1~1  SaveName=ScopeData26
  Trigonometric Function : Trigonometry  Operator=cos
  Trigonometric Function1 : Trigonometry  Operator=cos
  Trigonometric Function2 : Trigonometry  Operator=cos
  Trigonometric Function3 : Trigonometry
  Trigonometric Function4 : Trigonometry
  Trigonometric Function5 : Trigonometry
  Vdg : Outport
  Vqg : Outport  Port=2
  wires:
  Trigonometric Function1/1 -> Product2/1
  Constant/1 -> Add/2
  Trigonometric Function/1 -> Product1/1
  Trigonometric Function2/1 -> Product3/1
  Add/1 -> Trigonometric Function1/1
  Constant1/1 -> Add1/2
  Product2/1 -> Add2/2
  Product1/1 -> Add2/1
  Constant2/1 -> Add3/2
  Demux2/1 -> Product4/2, Product1/2
  Product5/1 -> Add5/2
  Constant3/1 -> Add4/2
  Add4/1 -> Trigonometric Function5/1
  Trigonometric Function3/1 -> Product4/1
  Trigonometric Function4/1 -> Product5/1
  Add3/1 -> Trigonometric Function4/1
  Trigonometric Function5/1 -> Product6/1
  Demux2/2 -> Product5/2, Product2/2
  Demux2/3 -> Product6/2, Product3/2
  Product4/1 -> Add5/1
  Add5/1 -> Gain1/1
  Product6/1 -> Add5/3
  Add1/1 -> Trigonometric Function2/1
  Product3/1 -> Add2/3
  Theta/1 -> Add/1, Trigonometric Function/1, Add1/1, Add4/1, Add3/1, Trigonometric Function3/1
  Vabc/1 -> Demux2/1
  Gain/1 -> Scope5/1, Vdg/1
  Add2/1 -> Gain/1
  Gain1/1 -> Scope5/2, Vqg/1

== system SVOC_DFIG/GSC Controller/abc//dq1 ==
  Iabc : Inport
  Theta : Inport  Port=2
  Add{,1,3..4} (4 alike) : Sum  Inputs=+-
  Add2 : Sum  Inputs=+++
  Add5 : Sum  Inputs=+++
  Constant : Constant  Value=(2*pi)/3
  Constant1 : Constant  Value=(4*pi)/3
  Constant2 : Constant  Value=(2*pi)/3
  Constant3 : Constant  Value=(4*pi)/3
  Demux2 : Demux  Outputs=3
  Gain : Gain  Gain=2/3
  Gain1 : Gain  Gain=-2/3
  Product{1..6} (6 alike) : Product
  Trigonometric Function : Trigonometry  Operator=cos
  Trigonometric Function1 : Trigonometry  Operator=cos
  Trigonometric Function2 : Trigonometry  Operator=cos
  Trigonometric Function3 : Trigonometry
  Trigonometric Function4 : Trigonometry
  Trigonometric Function5 : Trigonometry
  Idg : Outport
  Iqg : Outport  Port=2
  wires:
  Trigonometric Function1/1 -> Product2/1
  Constant/1 -> Add/2
  Trigonometric Function/1 -> Product1/1
  Trigonometric Function2/1 -> Product3/1
  Add/1 -> Trigonometric Function1/1
  Constant1/1 -> Add1/2
  Product2/1 -> Add2/2
  Product1/1 -> Add2/1
  Constant2/1 -> Add3/2
  Demux2/1 -> Product4/2, Product1/2
  Product5/1 -> Add5/2
  Constant3/1 -> Add4/2
  Add4/1 -> Trigonometric Function5/1
  Trigonometric Function3/1 -> Product4/1
  Trigonometric Function4/1 -> Product5/1
  Add3/1 -> Trigonometric Function4/1
  Trigonometric Function5/1 -> Product6/1
  Demux2/2 -> Product5/2, Product2/2
  Demux2/3 -> Product6/2, Product3/2
  Product4/1 -> Add5/1
  Add5/1 -> Gain1/1
  Product6/1 -> Add5/3
  Add1/1 -> Trigonometric Function2/1
  Product3/1 -> Add2/3
  Theta/1 -> Add/1, Trigonometric Function/1, Add1/1, Add4/1, Add3/1, Trigonometric Function3/1
  Gain1/1 -> Iqg/1
  Iabc/1 -> Demux2/1
  Gain/1 -> Idg/1
  Add2/1 -> Gain/1

== system SVOC_DFIG/GSC Controller/dq//abc ==
  vdq : Inport
  Theta : Inport  Port=2
  Add{,1..6} (7 alike) : Sum  Inputs=+-
  Constant : Constant  Value=(2*pi)/3
  Constant1 : Constant  Value=(4*pi)/3
  Constant2 : Constant  Value=(2*pi)/3
  Constant3 : Constant  Value=(4*pi)/3
  Demux2 : Demux  Outputs=2
  Product{1..6} (6 alike) : Product
  Trigonometric Function : Trigonometry  Operator=cos
  Trigonometric Function1 : Trigonometry  Operator=cos
  Trigonometric Function2 : Trigonometry  Operator=cos
  Trigonometric Function3 : Trigonometry
  Trigonometric Function4 : Trigonometry
  Trigonometric Function5 : Trigonometry
  Va : Outport
  Vb : Outport  Port=2
  Vc : Outport  Port=3
  wires:
  Trigonometric Function1/1 -> Product2/1
  Constant/1 -> Add/2
  Trigonometric Function/1 -> Product1/1
  Add/1 -> Trigonometric Function1/1
  Product1/1 -> Add2/1
  Constant2/1 -> Add3/2
  Demux2/1 -> Product1/2, Product2/2, Product3/2
  Trigonometric Function3/1 -> Product4/1
  Trigonometric Function4/1 -> Product5/1
  Add3/1 -> Trigonometric Function4/1
  vdq/1 -> Demux2/1
  Add2/1 -> Va/1
  Product4/1 -> Add2/2
  Demux2/2 -> Product4/2, Product6/2, Product5/2
  Product2/1 -> Add6/1
  Add6/1 -> Vb/1
  Product5/1 -> Add6/2
  Trigonometric Function2/1 -> Product3/1
  Constant1/1 -> Add1/2
  Add1/1 -> Trigonometric Function2/1
  Constant3/1 -> Add4/2
  Trigonometric Function5/1 -> Product6/1
  Add4/1 -> Trigonometric Function5/1
  Theta/1 -> Trigonometric Function/1, Trigonometric Function3/1, Add/1, Add4/1, Add1/1, Add3/1
  Product3/1 -> Add5/1
  Add5/1 -> Vc/1
  Product6/1 -> Add5/2

== system SVOC_DFIG/Grid/Grid Angle Detector ==
  Vabc_pu : Inport
  Add : Sum
  Beta1 : Fcn  Expr=(1/(3^.5))*(u(1)+2*u(2))
  Cartesian to Polar1 : simulink_extras/Transformations/Cartesian to Polar
  Constant : Constant  Value=2*pi
  Math Function : Math  Operator=rem  SaturateOnIntegerOverflow=on
  Scope5 : Scope
      settings: SaveName=ScopeData11
  alpha1 : Fcn  Expr=u(1)
  Grid Angle : Outport
  wires:
  Beta1/1 -> Cartesian to Polar1/2
  Vabc_pu/1 -> alpha1/1, Beta1/1
  Math Function/1 -> Grid Angle/1
  alpha1/1 -> Cartesian to Polar1/1
  Cartesian to Polar1/2 -> Add/1
  Constant/1 -> Math Function/2, Add/2
  Add/1 -> Math Function/1
  Cartesian to Polar1/1 -> Scope5/1

== system SVOC_DFIG/RSC Controller/abc//dq1 ==
  Irabc : Inport
  Theta_sl : Inport  Port=2
  Add{,1,3..4} (4 alike) : Sum  Inputs=+-
  Add2 : Sum  Inputs=+++
  Add5 : Sum  Inputs=+++
  Constant : Constant  Value=(2*pi)/3
  Constant1 : Constant  Value=(4*pi)/3
  Constant2 : Constant  Value=(2*pi)/3
  Constant3 : Constant  Value=(4*pi)/3
  Demux2 : Demux  Outputs=3
  Gain : Gain  Gain=2/3
  Gain1 : Gain  Gain=-2/3
  Product{1..6} (6 alike) : Product
  Trigonometric Function : Trigonometry  Operator=cos
  Trigonometric Function1 : Trigonometry  Operator=cos
  Trigonometric Function2 : Trigonometry  Operator=cos
  Trigonometric Function3 : Trigonometry
  Trigonometric Function4 : Trigonometry
  Trigonometric Function5 : Trigonometry
  Idr : Outport
  Iqr : Outport  Port=2
  wires:
  Trigonometric Function1/1 -> Product2/1
  Constant/1 -> Add/2
  Trigonometric Function/1 -> Product1/1
  Trigonometric Function2/1 -> Product3/1
  Add/1 -> Trigonometric Function1/1
  Constant1/1 -> Add1/2
  Product2/1 -> Add2/2
  Product1/1 -> Add2/1
  Constant2/1 -> Add3/2
  Demux2/1 -> Product4/2, Product1/2
  Product5/1 -> Add5/2
  Constant3/1 -> Add4/2
  Add4/1 -> Trigonometric Function5/1
  Trigonometric Function3/1 -> Product4/1
  Trigonometric Function4/1 -> Product5/1
  Add3/1 -> Trigonometric Function4/1
  Trigonometric Function5/1 -> Product6/1
  Demux2/2 -> Product5/2, Product2/2
  Demux2/3 -> Product6/2, Product3/2
  Product4/1 -> Add5/1
  Add5/1 -> Gain1/1
  Product6/1 -> Add5/3
  Add1/1 -> Trigonometric Function2/1
  Product3/1 -> Add2/3
  Theta_sl/1 -> Add/1, Trigonometric Function/1, Add1/1, Add4/1, Add3/1, Trigonometric Function3/1
  Gain1/1 -> Iqr/1
  Irabc/1 -> Demux2/1
  Gain/1 -> Idr/1
  Add2/1 -> Gain/1

== system SVOC_DFIG/RSC Controller/dq//abc ==
  vd_ref : Inport
  vq_ref : Inport  Port=2
  Theta_sl : Inport  Port=3
  Add{,1..6} (7 alike) : Sum  Inputs=+-
  Constant : Constant  Value=(2*pi)/3
  Constant1 : Constant  Value=(4*pi)/3
  Constant2 : Constant  Value=(2*pi)/3
  Constant3 : Constant  Value=(4*pi)/3
  Product{1..6} (6 alike) : Product
  Trigonometric Function : Trigonometry  Operator=cos
  Trigonometric Function1 : Trigonometry  Operator=cos
  Trigonometric Function2 : Trigonometry  Operator=cos
  Trigonometric Function3 : Trigonometry
  Trigonometric Function4 : Trigonometry
  Trigonometric Function5 : Trigonometry
  Var_ref : Outport
  Vbr_ref : Outport  Port=2
  Vcr_ref : Outport  Port=3
  wires:
  Trigonometric Function1/1 -> Product2/1
  Constant/1 -> Add/2
  Trigonometric Function/1 -> Product1/1
  Add/1 -> Trigonometric Function1/1
  Product1/1 -> Add2/1
  Constant2/1 -> Add3/2
  vd_ref/1 -> Product1/2, Product2/2, Product3/2
  Trigonometric Function3/1 -> Product4/1
  Trigonometric Function4/1 -> Product5/1
  Add3/1 -> Trigonometric Function4/1
  Add2/1 -> Var_ref/1
  Product4/1 -> Add2/2
  vq_ref/1 -> Product4/2, Product6/2, Product5/2
  Product2/1 -> Add6/1
  Add6/1 -> Vbr_ref/1
  Product5/1 -> Add6/2
  Trigonometric Function2/1 -> Product3/1
  Constant1/1 -> Add1/2
  Add1/1 -> Trigonometric Function2/1
  Constant3/1 -> Add4/2
  Trigonometric Function5/1 -> Product6/1
  Add4/1 -> Trigonometric Function5/1
  Theta_sl/1 -> Trigonometric Function/1, Trigonometric Function3/1, Add/1, Add4/1, Add1/1, Add3/1
  Product3/1 -> Add5/1
  Add5/1 -> Vcr_ref/1
  Product6/1 -> Add5/2

== system SVOC_DFIG/rSVM/Dwell Time Calculator ==
  Theta : Inport
  ma : Inport  Port=2
  Ts : Inport  Port=3
  Add : Sum  Inputs=--+
  Compare To Zero : simulink/Logic and Bit Operations/Compare To Zero  relop=>=  OutDataTypeStr=boolean
  Data Type Conversion : DataTypeConversion  OutDataTypeStr=double
  Mux : Mux  Inputs=3
  Product : Product  RndMeth=Zero
  Scope : Scope  NumInputPorts=3
      settings: YMin=0~0~-2.71051e-20  YMax=0.0001~0.0001~0.000425  SaveName=ScopeData12
  cTa : Fcn  Expr=u(2)*u(3)*sin((pi/3)-u(1))
  cTb : Fcn  Expr=u(2)*u(3)*sin(u(1))
  Ta : Outport
  Tb : Outport  Port=2
  T0 : Outport  Port=3
  wires:
  Product/1 -> Scope/1, T0/1
  Theta/1 -> Mux/1
  ma/1 -> Mux/2
  Ts/1 -> Add/3, Mux/3
  Mux/1 -> cTb/1, cTa/1
  Add/1 -> Product/2, Compare To Zero/1
  Data Type Conversion/1 -> Product/1
  Compare To Zero/1 -> Data Type Conversion/1
  cTa/1 -> Scope/2, Ta/1, Add/1
  cTb/1 -> Scope/3, Tb/1, Add/2

== system SVOC_DFIG/rSVM/Pulses ==
  Sector : Inport
  Ta1 : Inport  Port=2
  Tb1 : Inport  Port=3
  T0 : Inport  Port=4
  Data Type Conversion : DataTypeConversion  OutDataTypeStr=boolean
  Data Type Conversion1 : DataTypeConversion  OutDataTypeStr=boolean
  Data Type Conversion2 : DataTypeConversion  OutDataTypeStr=boolean
  Inverter Leg a : Subsystem
  Inverter Leg b : Subsystem
  Inverter Leg c : Subsystem
  Logical Operator : Logic  Operator=NOT  AllPortsSameDT=off
  Logical Operator1 : Logic  Operator=NOT  AllPortsSameDT=off
  Logical Operator2 : Logic  Operator=NOT  AllPortsSameDT=off
  Mux : Mux  Inputs=6
  Scope1 : Scope
      settings: SaveName=ScopeData2
  Scope3 : Scope
      settings: YMin=0  YMax=8  SaveName=ScopeData22
  Sector Select a : MultiPortSwitch  Inputs=6  DiagnosticForDefault=None
  Sector Select b : MultiPortSwitch  Inputs=6  DiagnosticForDefault=None
  Sector Select c : MultiPortSwitch  Inputs=6  DiagnosticForDefault=None
  Switching Segment Calculator : Subsystem
  Gating : Outport
  wires:
  Sector/1 -> Sector Select a/1, Scope1/1, Sector Select b/1, Sector Select c/1
  Data Type Conversion2/1 -> Logical Operator/1, Mux/1
  Data Type Conversion1/1 -> Logical Operator1/1, Mux/3
  Data Type Conversion/1 -> Logical Operator2/1, Mux/5
  Mux/1 -> Gating/1
  Logical Operator/1 -> Mux/2
  Logical Operator1/1 -> Mux/4
  Logical Operator2/1 -> Mux/6
  Switching Segment Calculator/1(Segment) -> Scope3/1, Inverter Leg c/1(Segment), Inverter Leg a/1(Segment), Inverter Leg b/1(Segment)
  T0/1 -> Switching Segment Calculator/1(T0)
  Ta1/1 -> Switching Segment Calculator/2(Ta)
  Tb1/1 -> Switching Segment Calculator/3(Tb)
  Inverter Leg a/1(Out1) -> Sector Select a/2
  Inverter Leg a/2(Out2) -> Sector Select a/3
  Inverter Leg a/3(Out3) -> Sector Select a/4
  Inverter Leg a/4(Out4) -> Sector Select a/5
  Inverter Leg a/5(Out5) -> Sector Select a/6
  Inverter Leg a/6(Out6) -> Sector Select a/7
  Inverter Leg b/1(Out1) -> Sector Select b/2
  Inverter Leg b/2(Out2) -> Sector Select b/3
  Inverter Leg b/3(Out3) -> Sector Select b/4
  Inverter Leg b/4(Out4) -> Sector Select b/5
  Inverter Leg b/5(Out5) -> Sector Select b/6
  Inverter Leg b/6(Out6) -> Sector Select b/7
  Inverter Leg c/1(Out1) -> Sector Select c/2
  Inverter Leg c/2(Out2) -> Sector Select c/3
  Inverter Leg c/3(Out3) -> Sector Select c/4
  Inverter Leg c/4(Out4) -> Sector Select c/5
  Inverter Leg c/5(Out5) -> Sector Select c/6
  Inverter Leg c/6(Out6) -> Sector Select c/7
  Sector Select c/1 -> Data Type Conversion/1
  Sector Select b/1 -> Data Type Conversion1/1
  Sector Select a/1 -> Data Type Conversion2/1

== system SVOC_DFIG/rSVM/Sector judge ==
  theta : Inport
  Add : Sum
  Constant : Constant  Value=2*pi
  Constant1 : Constant  OutDataTypeStr=boolean
  Constant2 : Constant  Value=2*pi
  Gain1 : Gain  Gain=3/pi
  Gain2 : Gain  Gain=pi/3
  Math Function1 : Math  Operator=rem  SaturateOnIntegerOverflow=on
  Rounding Function : Rounding
  Sum1 : Sum  Inputs=|++  SaturateOnIntegerOverflow=on
  Sum2 : Sum  Inputs=|-+
  Sector : Outport
  Cal_theta : Outport  Port=2
  wires:
  Gain1/1 -> Rounding Function/1
  Rounding Function/1 -> Gain2/1, Sum1/1
  Sum1/1 -> Sector/1
  Constant1/1 -> Sum1/2
  Gain2/1 -> Sum2/1
  Sum2/1 -> Cal_theta/1
  theta/1 -> Add/1
  Math Function1/1 -> Sum2/2, Gain1/1
  Constant/1 -> Add/2
  Add/1 -> Math Function1/1
  Constant2/1 -> Math Function1/2

== system SVOC_DFIG/rSVM/abc//alphabeta ==
  Vabc : Inport
  Beta1 : Fcn  Expr=(1/(3^.5))*(u(1)+2*u(2))
  alpha1 : Fcn  Expr=u(1)
  Valpha : Outport
  Vbeta : Outport  Port=2
  wires:
  Vabc/1 -> Beta1/1, alpha1/1
  alpha1/1 -> Valpha/1
  Beta1/1 -> Vbeta/1

== system SVOC_DFIG/sSVM/Dwell Time Calculator ==
  Theta : Inport
  ma : Inport  Port=2
  Ts : Inport  Port=3
  Add : Sum  Inputs=--+
  Compare To Zero : simulink/Logic and Bit Operations/Compare To Zero  relop=>=  OutDataTypeStr=boolean
  Data Type Conversion : DataTypeConversion  OutDataTypeStr=double
  Mux : Mux  Inputs=3
  Product : Product  RndMeth=Zero
  Scope : Scope  NumInputPorts=3
      settings: YMin=-5~-5~-5  YMax=5~5~5  SaveName=ScopeData12
  cTa : Fcn  Expr=u(2)*u(3)*sin((pi/3)-u(1))
  cTb : Fcn  Expr=u(2)*u(3)*sin(u(1))
  Ta : Outport
  Tb : Outport  Port=2
  T0 : Outport  Port=3
  wires:
  Product/1 -> Scope/1, T0/1
  Theta/1 -> Mux/1
  ma/1 -> Mux/2
  Ts/1 -> Add/3, Mux/3
  Mux/1 -> cTb/1, cTa/1
  Add/1 -> Product/2, Compare To Zero/1
  Data Type Conversion/1 -> Product/1
  Compare To Zero/1 -> Data Type Conversion/1
  cTa/1 -> Scope/2, Ta/1, Add/1
  cTb/1 -> Scope/3, Tb/1, Add/2

== system SVOC_DFIG/sSVM/Pulses ==
  Sector : Inport
  Ta1 : Inport  Port=2
  Tb1 : Inport  Port=3
  T0 : Inport  Port=4
  Data Type Conversion : DataTypeConversion  OutDataTypeStr=boolean
  Data Type Conversion1 : DataTypeConversion  OutDataTypeStr=boolean
  Data Type Conversion2 : DataTypeConversion  OutDataTypeStr=boolean
  Inverter Leg a : Subsystem
  Inverter Leg b : Subsystem
  Inverter Leg c : Subsystem
  Logical Operator : Logic  Operator=NOT  AllPortsSameDT=off
  Logical Operator1 : Logic  Operator=NOT  AllPortsSameDT=off
  Logical Operator2 : Logic  Operator=NOT  AllPortsSameDT=off
  Mux : Mux  Inputs=6
  Scope1 : Scope
      settings: SaveName=ScopeData2
  Scope3 : Scope
      settings: YMin=0  YMax=8  SaveName=ScopeData29
  Sector Select a : MultiPortSwitch  Inputs=6  DiagnosticForDefault=None
  Sector Select b : MultiPortSwitch  Inputs=6  DiagnosticForDefault=None
  Sector Select c : MultiPortSwitch  Inputs=6  DiagnosticForDefault=None
  Switching Segment Calculator : Subsystem
  Gating : Outport
  wires:
  Sector/1 -> Sector Select a/1, Scope1/1, Sector Select b/1, Sector Select c/1
  Data Type Conversion/1 -> Logical Operator/1, Mux/1
  Data Type Conversion1/1 -> Logical Operator1/1, Mux/3
  Data Type Conversion2/1 -> Logical Operator2/1, Mux/5
  Mux/1 -> Gating/1
  Logical Operator/1 -> Mux/2
  Logical Operator1/1 -> Mux/4
  Logical Operator2/1 -> Mux/6
  Switching Segment Calculator/1(Segment) -> Inverter Leg c/1(Segment), Inverter Leg a/1(Segment), Scope3/1, Inverter Leg b/1(Segment)
  T0/1 -> Switching Segment Calculator/1(T0)
  Ta1/1 -> Switching Segment Calculator/2(Ta)
  Tb1/1 -> Switching Segment Calculator/3(Tb)
  Inverter Leg a/1(Out1) -> Sector Select a/2
  Inverter Leg a/2(Out2) -> Sector Select a/3
  Inverter Leg a/3(Out3) -> Sector Select a/4
  Inverter Leg a/4(Out4) -> Sector Select a/5
  Inverter Leg a/5(Out5) -> Sector Select a/6
  Inverter Leg a/6(Out6) -> Sector Select a/7
  Inverter Leg b/1(Out1) -> Sector Select b/2
  Inverter Leg b/2(Out2) -> Sector Select b/3
  Inverter Leg b/3(Out3) -> Sector Select b/4
  Inverter Leg b/4(Out4) -> Sector Select b/5
  Inverter Leg b/5(Out5) -> Sector Select b/6
  Inverter Leg b/6(Out6) -> Sector Select b/7
  Inverter Leg c/1(Out1) -> Sector Select c/2
  Inverter Leg c/2(Out2) -> Sector Select c/3
  Inverter Leg c/3(Out3) -> Sector Select c/4
  Inverter Leg c/4(Out4) -> Sector Select c/5
  Inverter Leg c/5(Out5) -> Sector Select c/6
  Inverter Leg c/6(Out6) -> Sector Select c/7
  Sector Select a/1 -> Data Type Conversion/1
  Sector Select b/1 -> Data Type Conversion1/1
  Sector Select c/1 -> Data Type Conversion2/1

== system SVOC_DFIG/sSVM/Sector judge ==
  theta : Inport
  Add : Sum
  Constant : Constant  Value=2*pi
  Constant1 : Constant  OutDataTypeStr=boolean
  Constant2 : Constant  Value=2*pi
  Gain1 : Gain  Gain=3/pi
  Gain2 : Gain  Gain=pi/3
  Math Function1 : Math  Operator=rem  SaturateOnIntegerOverflow=on
  Rounding Function : Rounding
  Sum1 : Sum  Inputs=|++  SaturateOnIntegerOverflow=on
  Sum2 : Sum  Inputs=|-+
  Sector : Outport
  Cal_theta : Outport  Port=2
  wires:
  Gain1/1 -> Rounding Function/1
  Rounding Function/1 -> Gain2/1, Sum1/1
  Sum1/1 -> Sector/1
  Constant1/1 -> Sum1/2
  Gain2/1 -> Sum2/1
  Sum2/1 -> Cal_theta/1
  theta/1 -> Add/1
  Math Function1/1 -> Sum2/2, Gain1/1
  Constant/1 -> Add/2
  Add/1 -> Math Function1/1
  Constant2/1 -> Math Function1/2

== system SVOC_DFIG/sSVM/abc//alphabeta ==
  Vabc : Inport
  Beta1 : Fcn  Expr=(1/(3^.5))*(u(1)+2*u(2))
  alpha1 : Fcn  Expr=u(1)
  Valpha : Outport
  Vbeta : Outport  Port=2
  wires:
  Vabc/1 -> Beta1/1, alpha1/1
  alpha1/1 -> Valpha/1
  Beta1/1 -> Vbeta/1

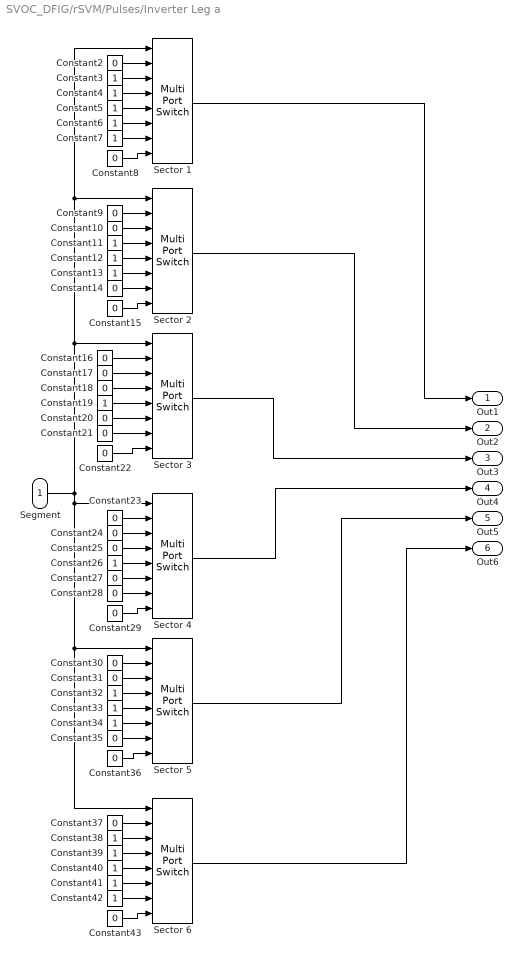
== system SVOC_DFIG/rSVM/Pulses/Inverter Leg a ==
  Segment : Inport
  Constant{2,8..10,14..18,20..25,27..31,35..37,43} (24 alike) : Constant  Value=0
  Constant{3..7,11..13,19,26,32..34,38..42} (18 alike) : Constant
  Sector {1..6} (6 alike) : MultiPortSwitch  Inputs=7
  Out1 : Outport
  Out2 : Outport  Port=2
  Out3 : Outport  Port=3
  Out4 : Outport  Port=4
  Out5 : Outport  Port=5
  Out6 : Outport  Port=6
  wires:
  Segment/1 -> Sector 6/1, Sector 5/1, Sector 4/1, Sector 2/1, Sector 1/1, Sector 3/1
  Sector 3/1 -> Out3/1
  Constant2/1 -> Sector 1/2
  Constant7/1 -> Sector 1/7
  Sector 1/1 -> Out1/1
  Constant3/1 -> Sector 1/3
  Constant6/1 -> Sector 1/6
  Constant10/1 -> Sector 2/3
  Sector 6/1 -> Out6/1
  Sector 2/1 -> Out2/1
  Constant5/1 -> Sector 1/5
  Constant9/1 -> Sector 2/2
  Constant4/1 -> Sector 1/4
  Constant8/1 -> Sector 1/8
  Sector 4/1 -> Out4/1
  Sector 5/1 -> Out5/1
  Constant42/1 -> Sector 6/7
  Constant43/1 -> Sector 6/8
  Constant40/1 -> Sector 6/5
  Constant37/1 -> Sector 6/2
  Constant41/1 -> Sector 6/6
  Constant39/1 -> Sector 6/4
  Constant17/1 -> Sector 3/3
  Constant30/1 -> Sector 5/2
  Constant38/1 -> Sector 6/3
  Constant29/1 -> Sector 4/8
  Constant28/1 -> Sector 4/7
  Constant31/1 -> Sector 5/3
  Constant25/1 -> Sector 4/4
  Constant20/1 -> Sector 3/6
  Constant26/1 -> Sector 4/5
  Constant32/1 -> Sector 5/4
  Constant33/1 -> Sector 5/5
  Constant36/1 -> Sector 5/8
  Constant18/1 -> Sector 3/4
  Constant14/1 -> Sector 2/7
  Constant13/1 -> Sector 2/6
  Constant34/1 -> Sector 5/6
  Constant24/1 -> Sector 4/3
  Constant11/1 -> Sector 2/4
  Constant16/1 -> Sector 3/2
  Constant21/1 -> Sector 3/7
  Constant12/1 -> Sector 2/5
  Constant19/1 -> Sector 3/5
  Constant35/1 -> Sector 5/7
  Constant22/1 -> Sector 3/8
  Constant23/1 -> Sector 4/2
  Constant15/1 -> Sector 2/8
  Constant27/1 -> Sector 4/6

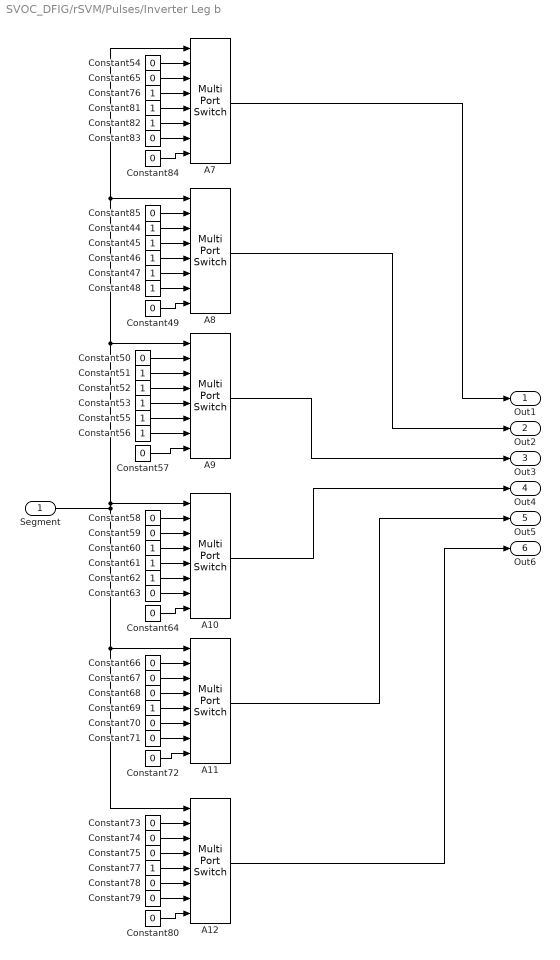
== system SVOC_DFIG/rSVM/Pulses/Inverter Leg b ==
  Segment : Inport
  A{7..12} (6 alike) : MultiPortSwitch  Inputs=7
  Constant{44..48,51..53,55..56,60..62,69,76..77,81..82} (18 alike) : Constant
  Constant{49..50,54,57..59,63..68,70..75,78..80,83..85} (24 alike) : Constant  Value=0
  Out1 : Outport
  Out2 : Outport  Port=2
  Out3 : Outport  Port=3
  Out4 : Outport  Port=4
  Out5 : Outport  Port=5
  Out6 : Outport  Port=6
  wires:
  Segment/1 -> A7/1, A8/1, A9/1, A10/1, A12/1, A11/1
  Constant80/1 -> A12/8
  Constant71/1 -> A11/7
  Constant69/1 -> A11/5
  Constant70/1 -> A11/6
  Constant72/1 -> A11/8
  Constant73/1 -> A12/2
  Constant75/1 -> A12/4
  Constant77/1 -> A12/5
  Constant79/1 -> A12/7
  Constant74/1 -> A12/3
  Constant68/1 -> A11/4
  Constant78/1 -> A12/6
  Constant55/1 -> A9/6
  Constant61/1 -> A10/5
  Constant47/1 -> A8/6
  Constant53/1 -> A9/5
  Constant45/1 -> A8/4
  Constant85/1 -> A8/2
  Constant49/1 -> A8/8
  Constant52/1 -> A9/4
  Constant56/1 -> A9/7
  Constant51/1 -> A9/3
  Constant57/1 -> A9/8
  Constant44/1 -> A8/3
  Constant46/1 -> A8/5
  Constant50/1 -> A9/2
  Constant48/1 -> A8/7
  Constant60/1 -> A10/4
  Constant62/1 -> A10/6
  Constant63/1 -> A10/7
  Constant64/1 -> A10/8
  Constant67/1 -> A11/3
  Constant66/1 -> A11/2
  Constant84/1 -> A7/8
  Constant59/1 -> A10/3
  Constant58/1 -> A10/2
  A9/1 -> Out3/1
  A8/1 -> Out2/1
  Constant65/1 -> A7/3
  A12/1 -> Out6/1
  A11/1 -> Out5/1
  A7/1 -> Out1/1
  Constant54/1 -> A7/2
  Constant76/1 -> A7/4
  A10/1 -> Out4/1
  Constant81/1 -> A7/5
  Constant82/1 -> A7/6
  Constant83/1 -> A7/7
